simulink model "MPHControl_1DoFSim"  (R2023b)
settings: Solver=VariableStepAuto  StartTime=0.0  StopTime=2  RelTol=1e-3
values from neighbouring files (symbols this model uses):
  alpha = Thrust_Moment    (= 14.2)    [init_1DoFSim.m]
  beta = Thrust_Moment    (= 14.2)    [init_1DoFSim.m]
  Inertia = [ .10 0 0 ... (first row only)    [init_1DoFSim.m]
  Moments = [0 0 0]    [init_1DoFSim.m]
  pqr_0 = [0 0 0]'    [init_1DoFSim.m]
  q_0 = Euler_To_Quaternion_ScalarFirst(Euler_Initial)'    [init_1DoFSim.m]
  q_desired = Euler_To_Quaternion_ScalarFirst(Euler_Desired)'    [init_1DoFSim.m]
  T = b/alpha - ((beta + alpha)*(alpha*b + b*beta - alpha*(((beta + alpha)*(- 2*beta*c + b^2 + 2*a*beta))/alpha)^(1/2)))/(alpha*(beta^2 + alpha*beta))    [init_1DoFSim.m]
  tau = -(alpha*b + b*beta - alpha*(((beta + alpha)*(- 2*beta*c + b^2 + 2*a*beta))/alpha)^(1/2))/(beta^2 + alpha*beta)    [init_1DoFSim.m]
libraries: aerolibanimutils x1, matrix_library x1, aerolibutil x1, vrlib x1
settings Model: Creator=benjackson  LastModifiedBy=ben
settings OptimizationCC: ReuseModelBlockBuffer=off

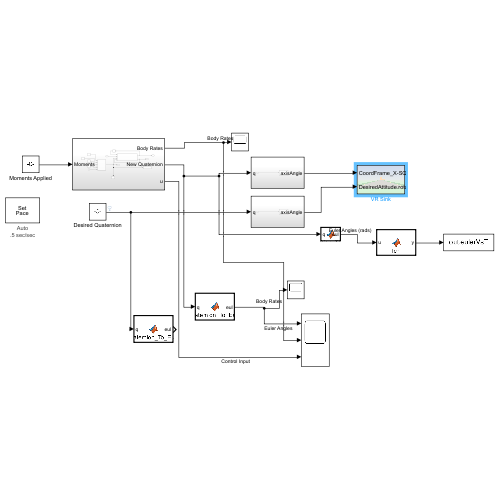
[thumbnail: Simulink's stored preview of the top-level diagram]
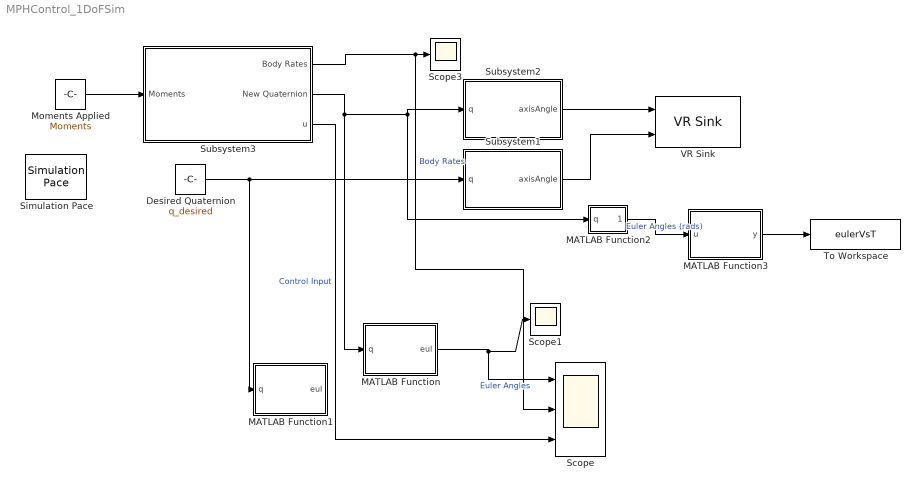
== system MPHControl_1DoFSim ==
  Desired Quaternion : Constant  Value=q_desired
  MATLAB Function : MATLAB Function  TreatAsAtomicUnit=on
  MATLAB Function1 : MATLAB Function  TreatAsAtomicUnit=on
  MATLAB Function2 : MATLAB Function  TreatAsAtomicUnit=on
  MATLAB Function3 : MATLAB Function  TreatAsAtomicUnit=on
  Moments Applied : Constant  Value=Moments
  Scope : Scope  NumInputPorts=3
  Scope1 : Scope
  Scope3 : Scope
  Simulation Pace : aerolibanimutils/Simulation Pace  SimulationPace=.5  SleepMode=Auto  OutputPaceError=off  SampleTime=1/100
  Subsystem1 : Subsystem
  Subsystem2 : Subsystem
  Subsystem3 : Subsystem
  To Workspace : ToWorkspace  VariableName=eulerVsT  SaveFormat=Timeseries  SampleTime=-1
  VR Sink : vrlib/VR Sink  InstantiateOnLoad=on  SampleTime=0.1  ViewEnable=on  RemoteChange=off  RemoteView=off  FieldsWritten=CoordFrame_X-SQUARE_Y-CIRCLE_Z-OCTOGO_Transform.rotation.4.1.1.double#DesiredAttitude.rotation.4.1.1.double  WorldFileName=World/World_RXN_WHL.x3d  WorldDescription=Straight Road Strip - 2 Lanes  AutoView=off  VideoDimensions=[]  AllowVariableSize=off
  wires:
  Moments Applied/1 -> Subsystem3/1(Moments)
  Subsystem3/2(New Quaternion) -> MATLAB Function2/1(q), Subsystem2/1(q), MATLAB Function/1(q)
  Subsystem3/1(Body Rates) -> Scope/2, Scope3/1  "Body Rates"
  Subsystem2/1(axisAngle) -> VR Sink/1
  Desired Quaternion/1 -> MATLAB Function1/1(q), Subsystem1/1(q)
  Subsystem1/1(axisAngle) -> VR Sink/2
  MATLAB Function/1(eul) -> Scope1/1, Scope/1  "Euler Angles"
  Subsystem3/3(u) -> Scope/3  "Control Input"
  MATLAB Function2/1(eul) -> MATLAB Function3/1(u)  "Euler Angles (rads)"
  MATLAB Function3/1(y) -> To Workspace/1

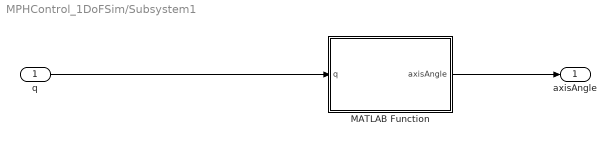
== system MPHControl_1DoFSim/Subsystem1 ==
  q : Inport
  MATLAB Function : MATLAB Function  TreatAsAtomicUnit=on
  axisAngle : Outport
  wires:
  q/1 -> MATLAB Function/1(q)
  MATLAB Function/1(axisAngle) -> axisAngle/1

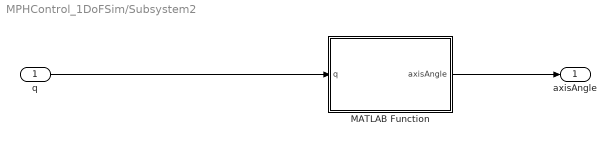
== system MPHControl_1DoFSim/Subsystem2 ==
  q : Inport
  MATLAB Function : MATLAB Function  TreatAsAtomicUnit=on
  axisAngle : Outport
  wires:
  q/1 -> MATLAB Function/1(q)
  MATLAB Function/1(axisAngle) -> axisAngle/1

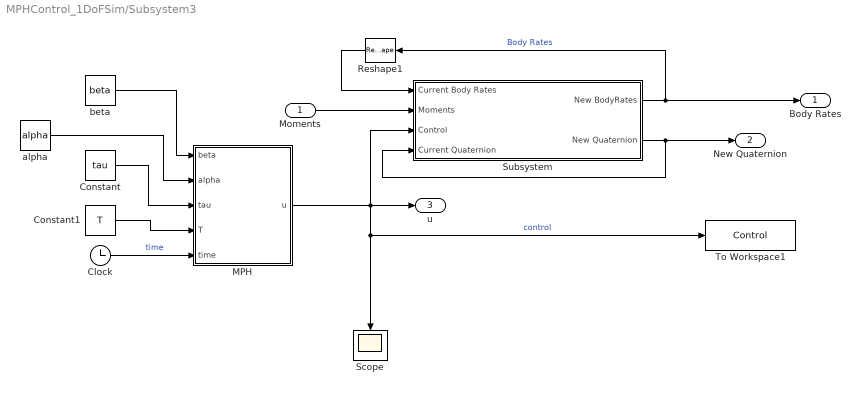
== system MPHControl_1DoFSim/Subsystem3 ==
  Moments : Inport
  Clock : Clock
  Constant : Constant  Value=tau
  Constant1 : Constant  Value=T
  MPH : MATLAB Function  TreatAsAtomicUnit=on
  Reshape1 : Reshape  OutputDimensionality=Customize  OutputDimensions=[1,3]
  Scope : Scope
  Subsystem : Subsystem
  To Workspace1 : ToWorkspace  VariableName=Control  SaveFormat=Timeseries  SampleTime=-1
  alpha : Constant  Value=alpha
  beta : Constant  Value=beta
  Body Rates : Outport
  New Quaternion : Outport  Port=2
  u : Outport  Port=3
  wires:
  Subsystem/1(New BodyRates) -> Reshape1/1, Body Rates/1  "Body Rates"
  Reshape1/1 -> Subsystem/1(Current Body Rates)
  Moments/1 -> Subsystem/2(Moments)
  MPH/1(u) -> u/1, Subsystem/3(Control), Scope/1, To Workspace1/1  "control"
  Subsystem/2(New Quaternion) -> New Quaternion/1, Subsystem/4(Current Quaternion)
  Constant/1 -> MPH/3(tau)
  Constant1/1 -> MPH/4(T)
  Clock/1 -> MPH/5(time)  "time"
  alpha/1 -> MPH/2(alpha)
  beta/1 -> MPH/1(beta)

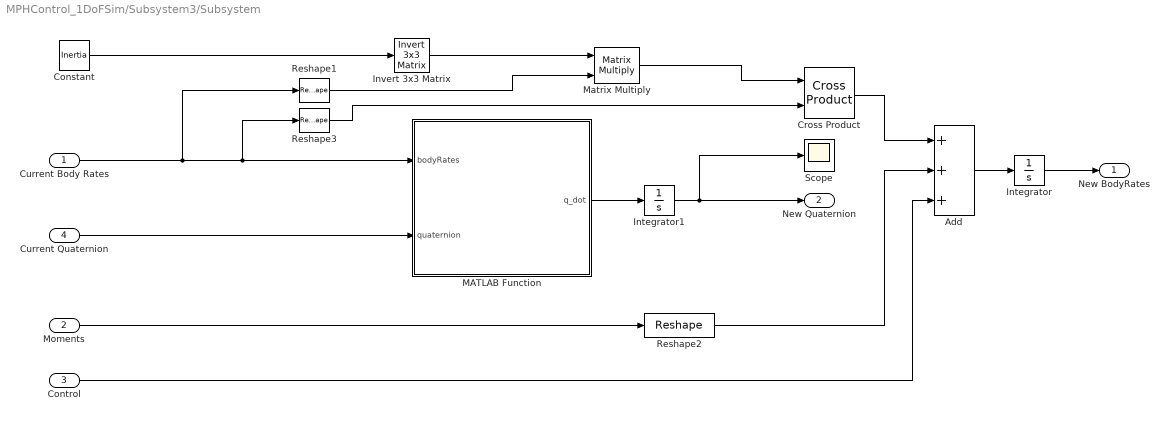
== system MPHControl_1DoFSim/Subsystem3/Subsystem ==
  Current Body Rates : Inport
  Moments : Inport  Port=2
  Control : Inport  Port=3
  Current Quaternion : Inport  Port=4
  Add : Sum  Inputs=+++
  Constant : Constant  Value=Inertia
  Cross Product : matrix_library/Cross Product
  Integrator : Integrator  InitialCondition=pqr_0
  Integrator1 : Integrator  InitialCondition=q_0
  Invert 3x3 Matrix : aerolibutil/Invert  3x3 Matrix
  MATLAB Function : MATLAB Function  TreatAsAtomicUnit=on
  Matrix Multiply : Product  Multiplication=Matrix(*)
  Reshape1 : Reshape  OutputDimensionality=Customize  OutputDimensions=[3,1]
  Reshape2 : Reshape  OutputDimensionality=Customize  OutputDimensions=[3,1]
  Reshape3 : Reshape  OutputDimensionality=Customize  OutputDimensions=[3,1]
  Scope : Scope
  New BodyRates : Outport
  New Quaternion : Outport  Port=2
  wires:
  Matrix Multiply/1 -> Cross Product/1
  Current Quaternion/1 -> MATLAB Function/2(quaternion)
  Integrator/1 -> New BodyRates/1
  Constant/1 -> Invert 3x3 Matrix/1
  MATLAB Function/1(q_dot) -> Integrator1/1
  Current Body Rates/1 -> Reshape1/1, Reshape3/1, MATLAB Function/1(bodyRates)
  Invert 3x3 Matrix/1 -> Matrix Multiply/1
  Cross Product/1 -> Add/1
  Add/1 -> Integrator/1
  Moments/1 -> Reshape2/1
  Reshape3/1 -> Cross Product/2
  Reshape1/1 -> Matrix Multiply/2
  Reshape2/1 -> Add/2
  Integrator1/1 -> Scope/1, New Quaternion/1
  Control/1 -> Add/3

== matlab function MPHControl_1DoFSim/Subsystem1/MATLAB Function ==
  data: q input; axisAngle output

function axisAngle = Quaternion_To_AxisAngle(q)
    for  i = 1:4
        if q(i) > 1 
            q(i) = 1.0;
            disp(q)
        end
    end

    qw = q(1);
    qx = q(2);
    qy = q(3);
    qz = q(4);
  

    theta = 2*acos(qw);

    if theta == 0 
        x = 1;
        y = 0;
        z = 0;
    else
        x = qx/(sin(theta/2));
        y = qy/(sin(theta/2));
        z = qz/(sin(theta/2));
    end
    
    %Vector comes first in our axis representation and angle comes last
    axisAngle = [x,z,y,theta];

end

== matlab function MPHControl_1DoFSim/Subsystem3/MPH ==
  data: beta input; alpha input; tau input; T input; time input; u output
function u = fcn(beta, alpha, tau,T, time)
    disp(time)
    if (time < tau)
        u = [beta 0 0]';
        disp("Fire")
    elseif (tau < time) && (time < T)
        u = [-alpha 0 0]';
    else
        u = [0 0 0]';
    end
end

== matlab function MPHControl_1DoFSim/MATLAB Function ==
  data: q input; eul output
function eul = Quaternion_To_Euler(q)
   
    qw = q(4);
    qx = q(1);
    qy = q(2);
    qz = q(3);
    q_mag = qw^2 +qx^2 +qy^2 +qz^2;
    
    q = q./q_mag;
    
    % Pre-allocate output
    eul = zeros(1, 3, 'like', q);
    
    % Cap all inputs to asin to 1, since values >1 produce complex
    % results
    % Since the quaternion is of unit length, this should never happen,
    % but some code generation configuration seem to hit this edge case
    % under some circumstances.
    aSinInput = -2*(qx.*qz-qw.*qy);
    mask1 = aSinInput >= 1 - 10*eps(class(qw));
    mask2 = aSinInput <= -1 + 10*eps(class(qw));
    aSinInput(mask1) = 1;
    aSinInput(mask2) = -1 ;
    mask = mask1 | mask2;
    
    eul = [ atan2( 2*(qx.*qy+qw.*qz), qw.^2 + qx.^2 - qy.^2 - qz.^2 ), ...
        asin( aSinInput ), ...
        atan2( 2*(qy.*qz+qw.*qx), qw.^2 - qx.^2 - qy.^2 + qz.^2 )];
    eul(mask, 1) = -sign(aSinInput(mask,1)).* 2 .* atan2(qx(mask,1), qw(mask,1));
    eul(mask, 3) = 0;
    
    % Check for complex numbers
    if ~isreal(eul)
        eul = real(eul);
    end
    
%     if nargout > 1
%         eul; % workaround for g2380983 (const folding heurstic issue during codegen)
%         eulAlt = robotics.core.internal.generateAlternateEulerAngles(eul, seq);
%     end
    
    
end

== matlab function MPHControl_1DoFSim/MATLAB Function1 ==
  data: q input; eul output
function eul = Quaternion_To_Euler(q)
   
    qw = q(4);
    qx = q(1);
    qy = q(2);
    qz = q(3);
    q_mag = qw^2 +qx^2 +qy^2 +qz^2;
    
    q = q./q_mag;
    
    % Pre-allocate output
    eul = zeros(1, 3, 'like', q);
    
    % Cap all inputs to asin to 1, since values >1 produce complex
    % results
    % Since the quaternion is of unit length, this should never happen,
    % but some code generation configuration seem to hit this edge case
    % under some circumstances.
    aSinInput = -2*(qx.*qz-qw.*qy);
    mask1 = aSinInput >= 1 - 10*eps(class(qw));
    mask2 = aSinInput <= -1 + 10*eps(class(qw));
    aSinInput(mask1) = 1;
    aSinInput(mask2) = -1 ;
    mask = mask1 | mask2;
    
    eul = [ atan2( 2*(qx.*qy+qw.*qz), qw.^2 + qx.^2 - qy.^2 - qz.^2 ), ...
        asin( aSinInput ), ...
        atan2( 2*(qy.*qz+qw.*qx), qw.^2 - qx.^2 - qy.^2 + qz.^2 )];
    eul(mask, 1) = -sign(aSinInput(mask,1)).* 2 .* atan2(qx(mask,1), qw(mask,1));
    eul(mask, 3) = 0;
    
    % Check for complex numbers
    if ~isreal(eul)
        eul = real(eul);
    end
    
%     if nargout > 1
%         eul; % workaround for g2380983 (const folding heurstic issue during codegen)
%         eulAlt = robotics.core.internal.generateAlternateEulerAngles(eul, seq);
%     end
    
    
end

== matlab function MPHControl_1DoFSim/Subsystem2/MATLAB Function ==
  data: q input; axisAngle output

function axisAngle = Quaternion_To_AxisAngle(q)
    for  i = 1:4
        if q(i) > 1 
            q(i) = 1.0;
            disp(q)
        end
    end

    qw = q(1);
    qx = q(2);
    qy = q(3);
    qz = q(4);
  

    theta = 2*acos(qw);

    if theta == 0 
        x = 1;
        y = 0;
        z = 0;
    else
        x = qx/(sin(theta/2));
        y = qy/(sin(theta/2));
        z = qz/(sin(theta/2));
    end
    
    %Vector comes first in our axis representation and angle comes last
    axisAngle = [x,z,y,theta];

end

== matlab function MPHControl_1DoFSim/MATLAB Function2 ==
  data: q input; eul output
function eul = Quaternion_To_Euler(q)
   
    qw = q(4);
    qx = q(1);
    qy = q(2);
    qz = q(3);
    q_mag = qw^2 +qx^2 +qy^2 +qz^2;
    
    q = q./q_mag;
    
    % Pre-allocate output
    eul = zeros(1, 3, 'like', q);
    
    % Cap all inputs to asin to 1, since values >1 produce complex
    % results
    % Since the quaternion is of unit length, this should never happen,
    % but some code generation configuration seem to hit this edge case
    % under some circumstances.
    aSinInput = -2*(qx.*qz-qw.*qy);
    mask1 = aSinInput >= 1 - 10*eps(class(qw));
    mask2 = aSinInput <= -1 + 10*eps(class(qw));
    aSinInput(mask1) = 1;
    aSinInput(mask2) = -1 ;
    mask = mask1 | mask2;
    
    eul = [ atan2( 2*(qx.*qy+qw.*qz), qw.^2 + qx.^2 - qy.^2 - qz.^2 ), ...
        asin( aSinInput ), ...
        atan2( 2*(qy.*qz+qw.*qx), qw.^2 - qx.^2 - qy.^2 + qz.^2 )];
    eul(mask, 1) = -sign(aSinInput(mask,1)).* 2 .* atan2(qx(mask,1), qw(mask,1));
    eul(mask, 3) = 0;
    
    % Check for complex numbers
    if ~isreal(eul)
        eul = real(eul);
    end
    
%     if nargout > 1
%         eul; % workaround for g2380983 (const folding heurstic issue during codegen)
%         eulAlt = robotics.core.internal.generateAlternateEulerAngles(eul, seq);
%     end
    
    
end

== matlab function MPHControl_1DoFSim/MATLAB Function3 ==
  data: u input; y output
function y = fcn(u)
    
y = u(1);

== matlab function MPHControl_1DoFSim/Subsystem3/Subsystem/MATLAB Function ==
  data: bodyRates input; quaternion input; q_dot output
function q_dot = getBodyRates(bodyRates,quaternion)

    p = bodyRates(1);
    q = bodyRates(2); 
    r = bodyRates(3);
    
    half_Q_Matrix =   0.5 * [  0, -p, -q, -r
                               p,  0,  r, -q
                               q, -r,  0,  p
                               r,  q, -p,  0];
                
    qVec  =  [quaternion(1); quaternion(2); quaternion(3); quaternion(4)];
    q_dot =  (half_Q_Matrix * qVec);     
    
end
